simulink model "elevatorMod"  (R2020a)
settings: Solver=VariableStepAuto  StartTime=0.0  StopTime=inf  RelTol=1e-3
PreLoadFcn:
  | slplc.api.loadDataTypes;
undefined symbols (not defined in the file): BOOL, DINT, INT, slplc
libraries: simulink x1
(part 4 of 39)

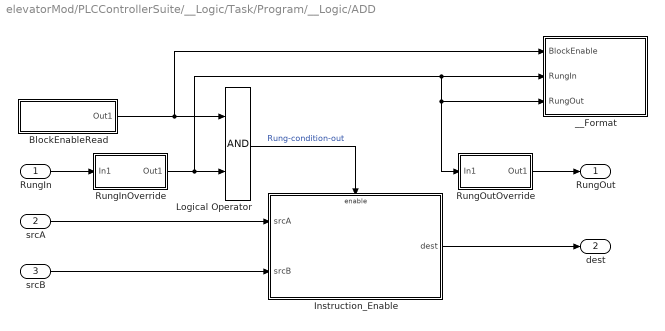
== system elevatorMod/PLCControllerSuite/__Logic/Task/Program/__Logic/ADD ==
  RungIn : Inport  OutDataTypeStr=BOOL  PortDimensions=1
  srcA : Inport  Port=2  PortDimensions=1
  srcB : Inport  Port=3  PortDimensions=1
  BlockEnableRead : Subsystem  DisableCoverage=on  TreatAsAtomicUnit=on  mask{PLCLabelTag=_Block_Enable, PLCBlockType=BlockEnableRead}
      mask prompts: PLCLabelTag "Label Tag:"
      mask init:
      | block = gcb;
      | maskObj = Simulink.Mask.get(block);
      | maskObj.Display = sprintf('disp(''%s'');', PLCLabelTag);
      mask Help: web([docroot '/plccoder/ref/blockenableread' '.html']);
      mask DialogControl PLCBlockTitle Prompt: Block Enable Read
      mask Display: disp('_Block_Enable');
  Instruction_Enable : Subsystem  TreatAsAtomicUnit=on
  Logical Operator : Logic  OutDataTypeStr=BOOL
  RungInOverride : Subsystem  DisableCoverage=on  TreatAsAtomicUnit=on
  RungOutOverride : Subsystem  DisableCoverage=on  TreatAsAtomicUnit=on
  __Format : MATLAB Function  Tag=PLC_Format_FC  Priority=20  DisableCoverage=on  InitFcn=slplc.utils.setBlockAppearance('reset');  StopFcn=slplc.utils.setBlockAppearance('reset');  TreatAsAtomicUnit=on
  RungOut : Outport  OutDataTypeStr=BOOL  PortDimensions=1  VectorParamsAs1DForOutWhenUnconnected=off
  dest : Outport  Port=2  PortDimensions=1  VectorParamsAs1DForOutWhenUnconnected=off
  wires:
  RungOutOverride/1(Out1) -> RungOut/1
  BlockEnableRead/1(Out1) -> __Format/1(BlockEnable), Logical Operator/1
  RungIn/1 -> RungInOverride/1(In1)
  RungInOverride/1(Out1) -> RungOutOverride/1(In1), __Format/3(RungOut), __Format/2(RungIn), Logical Operator/2
  srcA/1 -> Instruction_Enable/1(srcA)
  srcB/1 -> Instruction_Enable/2(srcB)
  Instruction_Enable/1(dest) -> dest/1
  Logical Operator/1 -> Instruction_Enable/Enable  "Rung-condition-out"

== system elevatorMod/PLCControllerSuite/__Logic/Task/Program/__Logic/Add Rungs ==

== system elevatorMod/PLCControllerSuite/__Logic/Task/Program/__Logic/Add Single Rung ==

== system elevatorMod/PLCControllerSuite/__Logic/Task/Program/__Logic/EQU ==
  RungIn : Inport  OutDataTypeStr=BOOL  PortDimensions=1
  srcA : Inport  Port=2  PortDimensions=1
  srcB : Inport  Port=3  PortDimensions=1
  BlockEnableRead : Subsystem  DisableCoverage=on  TreatAsAtomicUnit=on  mask{PLCLabelTag=_Block_Enable, PLCBlockType=BlockEnableRead}
      mask prompts: PLCLabelTag "Label Tag:"
      mask init:
      | block = gcb;
      | maskObj = Simulink.Mask.get(block);
      | maskObj.Display = sprintf('disp(''%s'');', PLCLabelTag);
      mask Help: web([docroot '/plccoder/ref/blockenableread' '.html']);
      mask DialogControl PLCBlockTitle Prompt: Block Enable Read
      mask Display: disp('_Block_Enable');
  Instruction_Enable : Subsystem  TreatAsAtomicUnit=on
  RungInOverride : Subsystem  DisableCoverage=on  TreatAsAtomicUnit=on
  __Format : MATLAB Function  Tag=PLC_Format_FC  Priority=20  DisableCoverage=on  InitFcn=slplc.utils.setBlockAppearance('reset');  StopFcn=slplc.utils.setBlockAppearance('reset');  TreatAsAtomicUnit=on
  RungOut : Outport  OutDataTypeStr=BOOL  PortDimensions=1  VectorParamsAs1DForOutWhenUnconnected=off
  wires:
  srcA/1 -> Instruction_Enable/2(srcA)
  Instruction_Enable/1(Rung-condition-out) -> RungOut/1, __Format/3(RungOut)
  srcB/1 -> Instruction_Enable/3(srcB)
  RungIn/1 -> RungInOverride/1(In1)
  RungInOverride/1(Out1) -> __Format/2(RungIn), Instruction_Enable/1(Rung-condition-in)
  BlockEnableRead/1(Out1) -> Instruction_Enable/Enable, __Format/1(BlockEnable)  "Rung-condition-out"

== system elevatorMod/PLCControllerSuite/__Logic/Task/Program/__Logic/EQU1 ==
  RungIn : Inport  OutDataTypeStr=BOOL  PortDimensions=1
  srcA : Inport  Port=2  PortDimensions=1
  srcB : Inport  Port=3  PortDimensions=1
  BlockEnableRead : Subsystem  DisableCoverage=on  TreatAsAtomicUnit=on  mask{PLCLabelTag=_Block_Enable, PLCBlockType=BlockEnableRead}
      mask prompts: PLCLabelTag "Label Tag:"
      mask init:
      | block = gcb;
      | maskObj = Simulink.Mask.get(block);
      | maskObj.Display = sprintf('disp(''%s'');', PLCLabelTag);
      mask Help: web([docroot '/plccoder/ref/blockenableread' '.html']);
      mask DialogControl PLCBlockTitle Prompt: Block Enable Read
      mask Display: disp('_Block_Enable');
  Instruction_Enable : Subsystem  TreatAsAtomicUnit=on
  RungInOverride : Subsystem  DisableCoverage=on  TreatAsAtomicUnit=on
  __Format : MATLAB Function  Tag=PLC_Format_FC  Priority=20  DisableCoverage=on  InitFcn=slplc.utils.setBlockAppearance('reset');  StopFcn=slplc.utils.setBlockAppearance('reset');  TreatAsAtomicUnit=on
  RungOut : Outport  OutDataTypeStr=BOOL  PortDimensions=1  VectorParamsAs1DForOutWhenUnconnected=off
  wires:
  BlockEnableRead/1(Out1) -> __Format/1(BlockEnable), Instruction_Enable/Enable  "Rung-condition-out"
  RungInOverride/1(Out1) -> Instruction_Enable/1(Rung-condition-in), __Format/2(RungIn)
  RungIn/1 -> RungInOverride/1(In1)
  srcB/1 -> Instruction_Enable/3(srcB)
  Instruction_Enable/1(Rung-condition-out) -> __Format/3(RungOut), RungOut/1
  srcA/1 -> Instruction_Enable/2(srcA)

== system elevatorMod/PLCControllerSuite/__Logic/Task/Program/__Logic/EQU2 ==
  RungIn : Inport  OutDataTypeStr=BOOL  PortDimensions=1
  srcA : Inport  Port=2  PortDimensions=1
  srcB : Inport  Port=3  PortDimensions=1
  BlockEnableRead : Subsystem  DisableCoverage=on  TreatAsAtomicUnit=on  mask{PLCLabelTag=_Block_Enable, PLCBlockType=BlockEnableRead}
      mask prompts: PLCLabelTag "Label Tag:"
      mask init:
      | block = gcb;
      | maskObj = Simulink.Mask.get(block);
      | maskObj.Display = sprintf('disp(''%s'');', PLCLabelTag);
      mask Help: web([docroot '/plccoder/ref/blockenableread' '.html']);
      mask DialogControl PLCBlockTitle Prompt: Block Enable Read
      mask Display: disp('_Block_Enable');
  Instruction_Enable : Subsystem  TreatAsAtomicUnit=on
  RungInOverride : Subsystem  DisableCoverage=on  TreatAsAtomicUnit=on
  __Format : MATLAB Function  Tag=PLC_Format_FC  Priority=20  DisableCoverage=on  InitFcn=slplc.utils.setBlockAppearance('reset');  StopFcn=slplc.utils.setBlockAppearance('reset');  TreatAsAtomicUnit=on
  RungOut : Outport  OutDataTypeStr=BOOL  PortDimensions=1  VectorParamsAs1DForOutWhenUnconnected=off
  wires:
  srcA/1 -> Instruction_Enable/2(srcA)
  Instruction_Enable/1(Rung-condition-out) -> RungOut/1, __Format/3(RungOut)
  srcB/1 -> Instruction_Enable/3(srcB)
  RungIn/1 -> RungInOverride/1(In1)
  RungInOverride/1(Out1) -> __Format/2(RungIn), Instruction_Enable/1(Rung-condition-in)
  BlockEnableRead/1(Out1) -> Instruction_Enable/Enable, __Format/1(BlockEnable)  "Rung-condition-out"

== system elevatorMod/PLCControllerSuite/__Logic/Task/Program/__Logic/EQU3 ==
  RungIn : Inport  OutDataTypeStr=BOOL  PortDimensions=1
  srcA : Inport  Port=2  PortDimensions=1
  srcB : Inport  Port=3  PortDimensions=1
  BlockEnableRead : Subsystem  DisableCoverage=on  TreatAsAtomicUnit=on  mask{PLCLabelTag=_Block_Enable, PLCBlockType=BlockEnableRead}
      mask prompts: PLCLabelTag "Label Tag:"
      mask init:
      | block = gcb;
      | maskObj = Simulink.Mask.get(block);
      | maskObj.Display = sprintf('disp(''%s'');', PLCLabelTag);
      mask Help: web([docroot '/plccoder/ref/blockenableread' '.html']);
      mask DialogControl PLCBlockTitle Prompt: Block Enable Read
      mask Display: disp('_Block_Enable');
  Instruction_Enable : Subsystem  TreatAsAtomicUnit=on
  RungInOverride : Subsystem  DisableCoverage=on  TreatAsAtomicUnit=on
  __Format : MATLAB Function  Tag=PLC_Format_FC  Priority=20  DisableCoverage=on  InitFcn=slplc.utils.setBlockAppearance('reset');  StopFcn=slplc.utils.setBlockAppearance('reset');  TreatAsAtomicUnit=on
  RungOut : Outport  OutDataTypeStr=BOOL  PortDimensions=1  VectorParamsAs1DForOutWhenUnconnected=off
  wires:
  srcA/1 -> Instruction_Enable/2(srcA)
  Instruction_Enable/1(Rung-condition-out) -> RungOut/1, __Format/3(RungOut)
  srcB/1 -> Instruction_Enable/3(srcB)
  RungIn/1 -> RungInOverride/1(In1)
  RungInOverride/1(Out1) -> __Format/2(RungIn), Instruction_Enable/1(Rung-condition-in)
  BlockEnableRead/1(Out1) -> Instruction_Enable/Enable, __Format/1(BlockEnable)  "Rung-condition-out"

== system elevatorMod/PLCControllerSuite/__Logic/Task/Program/__Logic/GRT ==
  RungIn : Inport  OutDataTypeStr=BOOL  PortDimensions=1
  srcA : Inport  Port=2  PortDimensions=1
  srcB : Inport  Port=3  PortDimensions=1
  BlockEnableRead : Subsystem  DisableCoverage=on  TreatAsAtomicUnit=on  mask{PLCLabelTag=_Block_Enable, PLCBlockType=BlockEnableRead}
      mask prompts: PLCLabelTag "Label Tag:"
      mask init:
      | block = gcb;
      | maskObj = Simulink.Mask.get(block);
      | maskObj.Display = sprintf('disp(''%s'');', PLCLabelTag);
      mask Help: web([docroot '/plccoder/ref/blockenableread' '.html']);
      mask DialogControl PLCBlockTitle Prompt: Block Enable Read
      mask Display: disp('_Block_Enable');
  Instruction_Enable : Subsystem  TreatAsAtomicUnit=on
  RungInOverride : Subsystem  DisableCoverage=on  TreatAsAtomicUnit=on
  __Format : MATLAB Function  Tag=PLC_Format_FC  Priority=20  DisableCoverage=on  InitFcn=slplc.utils.setBlockAppearance('reset');  StopFcn=slplc.utils.setBlockAppearance('reset');  TreatAsAtomicUnit=on
  RungOut : Outport  OutDataTypeStr=BOOL  PortDimensions=1  VectorParamsAs1DForOutWhenUnconnected=off
  wires:
  RungIn/1 -> RungInOverride/1(In1)
  srcB/1 -> Instruction_Enable/3(srcB)
  Instruction_Enable/1(Rung-condition-out) -> RungOut/1, __Format/3(RungOut)
  BlockEnableRead/1(Out1) -> Instruction_Enable/Enable, __Format/1(BlockEnable)
  RungInOverride/1(Out1) -> Instruction_Enable/1(Rung-condition-in), __Format/2(RungIn)
  srcA/1 -> Instruction_Enable/2(srcA)

== system elevatorMod/PLCControllerSuite/__Logic/Task/Program/__Logic/Junction ==
  RungIn1 : Inport
  RungIn2 : Inport  Port=2
  BlockEnableRead : Subsystem  DisableCoverage=on  TreatAsAtomicUnit=on  mask{PLCLabelTag=_Block_Enable, PLCBlockType=BlockEnableRead}
      mask prompts: PLCLabelTag "Label Tag:"
      mask init:
      | block = gcb;
      | maskObj = Simulink.Mask.get(block);
      | maskObj.Display = sprintf('disp(''%s'');', PLCLabelTag);
      mask Help: web([docroot '/plccoder/ref/blockenableread' '.html']);
      mask DialogControl PLCBlockTitle Prompt: Block Enable Read
      mask Display: disp('_Block_Enable');
  __Enable : Subsystem  TreatAsAtomicUnit=on
  __Format : MATLAB Function  Tag=PLC_Format_Joint  Priority=20  DisableCoverage=on  InitFcn=slplc.utils.setBlockAppearance('reset', '', {'black', 'black'});  StopFcn=slplc.utils.setBlockAppearance('reset', '', {'black', 'black'});  TreatAsAtomicUnit=on
  RungOut : Outport  VectorParamsAs1DForOutWhenUnconnected=off
  wires:
  __Enable/1(RungOut) -> RungOut/1, __Format/2(RungOut)
  RungIn2/1 -> __Enable/2(RungIn2)
  RungIn1/1 -> __Enable/1(RungIn1)
  BlockEnableRead/1(Out1) -> __Enable/Enable, __Format/1(BlockEnable)

== system elevatorMod/PLCControllerSuite/__Logic/Task/Program/__Logic/Junction1 ==
  RungIn1 : Inport
  RungIn2 : Inport  Port=2
  BlockEnableRead : Subsystem  DisableCoverage=on  TreatAsAtomicUnit=on  mask{PLCLabelTag=_Block_Enable, PLCBlockType=BlockEnableRead}
      mask prompts: PLCLabelTag "Label Tag:"
      mask init:
      | block = gcb;
      | maskObj = Simulink.Mask.get(block);
      | maskObj.Display = sprintf('disp(''%s'');', PLCLabelTag);
      mask Help: web([docroot '/plccoder/ref/blockenableread' '.html']);
      mask DialogControl PLCBlockTitle Prompt: Block Enable Read
      mask Display: disp('_Block_Enable');
  __Enable : Subsystem  TreatAsAtomicUnit=on
  __Format : MATLAB Function  Tag=PLC_Format_Joint  Priority=20  DisableCoverage=on  InitFcn=slplc.utils.setBlockAppearance('reset', '', {'black', 'black'});  StopFcn=slplc.utils.setBlockAppearance('reset', '', {'black', 'black'});  TreatAsAtomicUnit=on
  RungOut : Outport  VectorParamsAs1DForOutWhenUnconnected=off
  wires:
  BlockEnableRead/1(Out1) -> __Format/1(BlockEnable), __Enable/Enable
  RungIn1/1 -> __Enable/1(RungIn1)
  RungIn2/1 -> __Enable/2(RungIn2)
  __Enable/1(RungOut) -> __Format/2(RungOut), RungOut/1

== system elevatorMod/PLCControllerSuite/__Logic/Task/Program/__Logic/Junction10 ==
  RungIn1 : Inport
  RungIn2 : Inport  Port=2
  BlockEnableRead : Subsystem  DisableCoverage=on  TreatAsAtomicUnit=on  mask{PLCLabelTag=_Block_Enable, PLCBlockType=BlockEnableRead}
      mask prompts: PLCLabelTag "Label Tag:"
      mask init:
      | block = gcb;
      | maskObj = Simulink.Mask.get(block);
      | maskObj.Display = sprintf('disp(''%s'');', PLCLabelTag);
      mask Help: web([docroot '/plccoder/ref/blockenableread' '.html']);
      mask DialogControl PLCBlockTitle Prompt: Block Enable Read
      mask Display: disp('_Block_Enable');
  __Enable : Subsystem  TreatAsAtomicUnit=on
  __Format : MATLAB Function  Tag=PLC_Format_Joint  Priority=20  DisableCoverage=on  InitFcn=slplc.utils.setBlockAppearance('reset', '', {'black', 'black'});  StopFcn=slplc.utils.setBlockAppearance('reset', '', {'black', 'black'});  TreatAsAtomicUnit=on
  RungOut : Outport  VectorParamsAs1DForOutWhenUnconnected=off
  wires:
  __Enable/1(RungOut) -> RungOut/1, __Format/2(RungOut)
  RungIn2/1 -> __Enable/2(RungIn2)
  RungIn1/1 -> __Enable/1(RungIn1)
  BlockEnableRead/1(Out1) -> __Enable/Enable, __Format/1(BlockEnable)

== system elevatorMod/PLCControllerSuite/__Logic/Task/Program/__Logic/Junction11 ==
  RungIn1 : Inport
  RungIn2 : Inport  Port=2
  BlockEnableRead : Subsystem  DisableCoverage=on  TreatAsAtomicUnit=on  mask{PLCLabelTag=_Block_Enable, PLCBlockType=BlockEnableRead}
      mask prompts: PLCLabelTag "Label Tag:"
      mask init:
      | block = gcb;
      | maskObj = Simulink.Mask.get(block);
      | maskObj.Display = sprintf('disp(''%s'');', PLCLabelTag);
      mask Help: web([docroot '/plccoder/ref/blockenableread' '.html']);
      mask DialogControl PLCBlockTitle Prompt: Block Enable Read
      mask Display: disp('_Block_Enable');
  __Enable : Subsystem  TreatAsAtomicUnit=on
  __Format : MATLAB Function  Tag=PLC_Format_Joint  Priority=20  DisableCoverage=on  InitFcn=slplc.utils.setBlockAppearance('reset', '', {'black', 'black'});  StopFcn=slplc.utils.setBlockAppearance('reset', '', {'black', 'black'});  TreatAsAtomicUnit=on
  RungOut : Outport  VectorParamsAs1DForOutWhenUnconnected=off
  wires:
  __Enable/1(RungOut) -> RungOut/1, __Format/2(RungOut)
  RungIn2/1 -> __Enable/2(RungIn2)
  RungIn1/1 -> __Enable/1(RungIn1)
  BlockEnableRead/1(Out1) -> __Enable/Enable, __Format/1(BlockEnable)

== system elevatorMod/PLCControllerSuite/__Logic/Task/Program/__Logic/Junction12 ==
  RungIn1 : Inport
  RungIn2 : Inport  Port=2
  BlockEnableRead : Subsystem  DisableCoverage=on  TreatAsAtomicUnit=on  mask{PLCLabelTag=_Block_Enable, PLCBlockType=BlockEnableRead}
      mask prompts: PLCLabelTag "Label Tag:"
      mask init:
      | block = gcb;
      | maskObj = Simulink.Mask.get(block);
      | maskObj.Display = sprintf('disp(''%s'');', PLCLabelTag);
      mask Help: web([docroot '/plccoder/ref/blockenableread' '.html']);
      mask DialogControl PLCBlockTitle Prompt: Block Enable Read
      mask Display: disp('_Block_Enable');
  __Enable : Subsystem  TreatAsAtomicUnit=on
  __Format : MATLAB Function  Tag=PLC_Format_Joint  Priority=20  DisableCoverage=on  InitFcn=slplc.utils.setBlockAppearance('reset', '', {'black', 'black'});  StopFcn=slplc.utils.setBlockAppearance('reset', '', {'black', 'black'});  TreatAsAtomicUnit=on
  RungOut : Outport  VectorParamsAs1DForOutWhenUnconnected=off
  wires:
  BlockEnableRead/1(Out1) -> __Format/1(BlockEnable), __Enable/Enable
  RungIn1/1 -> __Enable/1(RungIn1)
  RungIn2/1 -> __Enable/2(RungIn2)
  __Enable/1(RungOut) -> __Format/2(RungOut), RungOut/1

== system elevatorMod/PLCControllerSuite/__Logic/Task/Program/__Logic/Junction13 ==
  RungIn1 : Inport
  RungIn2 : Inport  Port=2
  BlockEnableRead : Subsystem  DisableCoverage=on  TreatAsAtomicUnit=on  mask{PLCLabelTag=_Block_Enable, PLCBlockType=BlockEnableRead}
      mask prompts: PLCLabelTag "Label Tag:"
      mask init:
      | block = gcb;
      | maskObj = Simulink.Mask.get(block);
      | maskObj.Display = sprintf('disp(''%s'');', PLCLabelTag);
      mask Help: web([docroot '/plccoder/ref/blockenableread' '.html']);
      mask DialogControl PLCBlockTitle Prompt: Block Enable Read
      mask Display: disp('_Block_Enable');
  __Enable : Subsystem  TreatAsAtomicUnit=on
  __Format : MATLAB Function  Tag=PLC_Format_Joint  Priority=20  DisableCoverage=on  InitFcn=slplc.utils.setBlockAppearance('reset', '', {'black', 'black'});  StopFcn=slplc.utils.setBlockAppearance('reset', '', {'black', 'black'});  TreatAsAtomicUnit=on
  RungOut : Outport  VectorParamsAs1DForOutWhenUnconnected=off
  wires:
  __Enable/1(RungOut) -> RungOut/1, __Format/2(RungOut)
  RungIn2/1 -> __Enable/2(RungIn2)
  RungIn1/1 -> __Enable/1(RungIn1)
  BlockEnableRead/1(Out1) -> __Enable/Enable, __Format/1(BlockEnable)

== system elevatorMod/PLCControllerSuite/__Logic/Task/Program/__Logic/Junction14 ==
  RungIn1 : Inport
  RungIn2 : Inport  Port=2
  BlockEnableRead : Subsystem  DisableCoverage=on  TreatAsAtomicUnit=on  mask{PLCLabelTag=_Block_Enable, PLCBlockType=BlockEnableRead}
      mask prompts: PLCLabelTag "Label Tag:"
      mask init:
      | block = gcb;
      | maskObj = Simulink.Mask.get(block);
      | maskObj.Display = sprintf('disp(''%s'');', PLCLabelTag);
      mask Help: web([docroot '/plccoder/ref/blockenableread' '.html']);
      mask DialogControl PLCBlockTitle Prompt: Block Enable Read
      mask Display: disp('_Block_Enable');
  __Enable : Subsystem  TreatAsAtomicUnit=on
  __Format : MATLAB Function  Tag=PLC_Format_Joint  Priority=20  DisableCoverage=on  InitFcn=slplc.utils.setBlockAppearance('reset', '', {'black', 'black'});  StopFcn=slplc.utils.setBlockAppearance('reset', '', {'black', 'black'});  TreatAsAtomicUnit=on
  RungOut : Outport  VectorParamsAs1DForOutWhenUnconnected=off
  wires:
  BlockEnableRead/1(Out1) -> __Format/1(BlockEnable), __Enable/Enable
  RungIn1/1 -> __Enable/1(RungIn1)
  RungIn2/1 -> __Enable/2(RungIn2)
  __Enable/1(RungOut) -> __Format/2(RungOut), RungOut/1

== system elevatorMod/PLCControllerSuite/__Logic/Task/Program/__Logic/Junction15 ==
  RungIn1 : Inport
  RungIn2 : Inport  Port=2
  BlockEnableRead : Subsystem  DisableCoverage=on  TreatAsAtomicUnit=on  mask{PLCLabelTag=_Block_Enable, PLCBlockType=BlockEnableRead}
      mask prompts: PLCLabelTag "Label Tag:"
      mask init:
      | block = gcb;
      | maskObj = Simulink.Mask.get(block);
      | maskObj.Display = sprintf('disp(''%s'');', PLCLabelTag);
      mask Help: web([docroot '/plccoder/ref/blockenableread' '.html']);
      mask DialogControl PLCBlockTitle Prompt: Block Enable Read
      mask Display: disp('_Block_Enable');
  __Enable : Subsystem  TreatAsAtomicUnit=on
  __Format : MATLAB Function  Tag=PLC_Format_Joint  Priority=20  DisableCoverage=on  InitFcn=slplc.utils.setBlockAppearance('reset', '', {'black', 'black'});  StopFcn=slplc.utils.setBlockAppearance('reset', '', {'black', 'black'});  TreatAsAtomicUnit=on
  RungOut : Outport  VectorParamsAs1DForOutWhenUnconnected=off
  wires:
  __Enable/1(RungOut) -> RungOut/1, __Format/2(RungOut)
  RungIn2/1 -> __Enable/2(RungIn2)
  RungIn1/1 -> __Enable/1(RungIn1)
  BlockEnableRead/1(Out1) -> __Enable/Enable, __Format/1(BlockEnable)

== system elevatorMod/PLCControllerSuite/__Logic/Task/Program/__Logic/Junction16 ==
  RungIn1 : Inport
  RungIn2 : Inport  Port=2
  BlockEnableRead : Subsystem  DisableCoverage=on  TreatAsAtomicUnit=on  mask{PLCLabelTag=_Block_Enable, PLCBlockType=BlockEnableRead}
      mask prompts: PLCLabelTag "Label Tag:"
      mask init:
      | block = gcb;
      | maskObj = Simulink.Mask.get(block);
      | maskObj.Display = sprintf('disp(''%s'');', PLCLabelTag);
      mask Help: web([docroot '/plccoder/ref/blockenableread' '.html']);
      mask DialogControl PLCBlockTitle Prompt: Block Enable Read
      mask Display: disp('_Block_Enable');
  __Enable : Subsystem  TreatAsAtomicUnit=on
  __Format : MATLAB Function  Tag=PLC_Format_Joint  Priority=20  DisableCoverage=on  InitFcn=slplc.utils.setBlockAppearance('reset', '', {'black', 'black'});  StopFcn=slplc.utils.setBlockAppearance('reset', '', {'black', 'black'});  TreatAsAtomicUnit=on
  RungOut : Outport  VectorParamsAs1DForOutWhenUnconnected=off
  wires:
  BlockEnableRead/1(Out1) -> __Format/1(BlockEnable), __Enable/Enable
  RungIn1/1 -> __Enable/1(RungIn1)
  RungIn2/1 -> __Enable/2(RungIn2)
  __Enable/1(RungOut) -> __Format/2(RungOut), RungOut/1

== system elevatorMod/PLCControllerSuite/__Logic/Task/Program/__Logic/Junction17 ==
  RungIn1 : Inport
  RungIn2 : Inport  Port=2
  BlockEnableRead : Subsystem  DisableCoverage=on  TreatAsAtomicUnit=on  mask{PLCLabelTag=_Block_Enable, PLCBlockType=BlockEnableRead}
      mask prompts: PLCLabelTag "Label Tag:"
      mask init:
      | block = gcb;
      | maskObj = Simulink.Mask.get(block);
      | maskObj.Display = sprintf('disp(''%s'');', PLCLabelTag);
      mask Help: web([docroot '/plccoder/ref/blockenableread' '.html']);
      mask DialogControl PLCBlockTitle Prompt: Block Enable Read
      mask Display: disp('_Block_Enable');
  __Enable : Subsystem  TreatAsAtomicUnit=on
  __Format : MATLAB Function  Tag=PLC_Format_Joint  Priority=20  DisableCoverage=on  InitFcn=slplc.utils.setBlockAppearance('reset', '', {'black', 'black'});  StopFcn=slplc.utils.setBlockAppearance('reset', '', {'black', 'black'});  TreatAsAtomicUnit=on
  RungOut : Outport  VectorParamsAs1DForOutWhenUnconnected=off
  wires:
  __Enable/1(RungOut) -> RungOut/1, __Format/2(RungOut)
  RungIn2/1 -> __Enable/2(RungIn2)
  RungIn1/1 -> __Enable/1(RungIn1)
  BlockEnableRead/1(Out1) -> __Enable/Enable, __Format/1(BlockEnable)

== system elevatorMod/PLCControllerSuite/__Logic/Task/Program/__Logic/Junction18 ==
  RungIn1 : Inport
  RungIn2 : Inport  Port=2
  BlockEnableRead : Subsystem  DisableCoverage=on  TreatAsAtomicUnit=on  mask{PLCLabelTag=_Block_Enable, PLCBlockType=BlockEnableRead}
      mask prompts: PLCLabelTag "Label Tag:"
      mask init:
      | block = gcb;
      | maskObj = Simulink.Mask.get(block);
      | maskObj.Display = sprintf('disp(''%s'');', PLCLabelTag);
      mask Help: web([docroot '/plccoder/ref/blockenableread' '.html']);
      mask DialogControl PLCBlockTitle Prompt: Block Enable Read
      mask Display: disp('_Block_Enable');
  __Enable : Subsystem  TreatAsAtomicUnit=on
  __Format : MATLAB Function  Tag=PLC_Format_Joint  Priority=20  DisableCoverage=on  InitFcn=slplc.utils.setBlockAppearance('reset', '', {'black', 'black'});  StopFcn=slplc.utils.setBlockAppearance('reset', '', {'black', 'black'});  TreatAsAtomicUnit=on
  RungOut : Outport  VectorParamsAs1DForOutWhenUnconnected=off
  wires:
  __Enable/1(RungOut) -> RungOut/1, __Format/2(RungOut)
  RungIn2/1 -> __Enable/2(RungIn2)
  RungIn1/1 -> __Enable/1(RungIn1)
  BlockEnableRead/1(Out1) -> __Enable/Enable, __Format/1(BlockEnable)

== system elevatorMod/PLCControllerSuite/__Logic/Task/Program/__Logic/Junction19 ==
  RungIn1 : Inport
  RungIn2 : Inport  Port=2
  BlockEnableRead : Subsystem  DisableCoverage=on  TreatAsAtomicUnit=on  mask{PLCLabelTag=_Block_Enable, PLCBlockType=BlockEnableRead}
      mask prompts: PLCLabelTag "Label Tag:"
      mask init:
      | block = gcb;
      | maskObj = Simulink.Mask.get(block);
      | maskObj.Display = sprintf('disp(''%s'');', PLCLabelTag);
      mask Help: web([docroot '/plccoder/ref/blockenableread' '.html']);
      mask DialogControl PLCBlockTitle Prompt: Block Enable Read
      mask Display: disp('_Block_Enable');
  __Enable : Subsystem  TreatAsAtomicUnit=on
  __Format : MATLAB Function  Tag=PLC_Format_Joint  Priority=20  DisableCoverage=on  InitFcn=slplc.utils.setBlockAppearance('reset', '', {'black', 'black'});  StopFcn=slplc.utils.setBlockAppearance('reset', '', {'black', 'black'});  TreatAsAtomicUnit=on
  RungOut : Outport  VectorParamsAs1DForOutWhenUnconnected=off
  wires:
  __Enable/1(RungOut) -> RungOut/1, __Format/2(RungOut)
  RungIn2/1 -> __Enable/2(RungIn2)
  RungIn1/1 -> __Enable/1(RungIn1)
  BlockEnableRead/1(Out1) -> __Enable/Enable, __Format/1(BlockEnable)

== system elevatorMod/PLCControllerSuite/__Logic/Task/Program/__Logic/Junction2 ==
  RungIn1 : Inport
  RungIn2 : Inport  Port=2
  BlockEnableRead : Subsystem  DisableCoverage=on  TreatAsAtomicUnit=on  mask{PLCLabelTag=_Block_Enable, PLCBlockType=BlockEnableRead}
      mask prompts: PLCLabelTag "Label Tag:"
      mask init:
      | block = gcb;
      | maskObj = Simulink.Mask.get(block);
      | maskObj.Display = sprintf('disp(''%s'');', PLCLabelTag);
      mask Help: web([docroot '/plccoder/ref/blockenableread' '.html']);
      mask DialogControl PLCBlockTitle Prompt: Block Enable Read
      mask Display: disp('_Block_Enable');
  __Enable : Subsystem  TreatAsAtomicUnit=on
  __Format : MATLAB Function  Tag=PLC_Format_Joint  Priority=20  DisableCoverage=on  InitFcn=slplc.utils.setBlockAppearance('reset', '', {'black', 'black'});  StopFcn=slplc.utils.setBlockAppearance('reset', '', {'black', 'black'});  TreatAsAtomicUnit=on
  RungOut : Outport  VectorParamsAs1DForOutWhenUnconnected=off
  wires:
  __Enable/1(RungOut) -> RungOut/1, __Format/2(RungOut)
  RungIn2/1 -> __Enable/2(RungIn2)
  RungIn1/1 -> __Enable/1(RungIn1)
  BlockEnableRead/1(Out1) -> __Enable/Enable, __Format/1(BlockEnable)

== system elevatorMod/PLCControllerSuite/__Logic/Task/Program/__Logic/Junction20 ==
  RungIn1 : Inport
  RungIn2 : Inport  Port=2
  BlockEnableRead : Subsystem  DisableCoverage=on  TreatAsAtomicUnit=on  mask{PLCLabelTag=_Block_Enable, PLCBlockType=BlockEnableRead}
      mask prompts: PLCLabelTag "Label Tag:"
      mask init:
      | block = gcb;
      | maskObj = Simulink.Mask.get(block);
      | maskObj.Display = sprintf('disp(''%s'');', PLCLabelTag);
      mask Help: web([docroot '/plccoder/ref/blockenableread' '.html']);
      mask DialogControl PLCBlockTitle Prompt: Block Enable Read
      mask Display: disp('_Block_Enable');
  __Enable : Subsystem  TreatAsAtomicUnit=on
  __Format : MATLAB Function  Tag=PLC_Format_Joint  Priority=20  DisableCoverage=on  InitFcn=slplc.utils.setBlockAppearance('reset', '', {'black', 'black'});  StopFcn=slplc.utils.setBlockAppearance('reset', '', {'black', 'black'});  TreatAsAtomicUnit=on
  RungOut : Outport  VectorParamsAs1DForOutWhenUnconnected=off
  wires:
  __Enable/1(RungOut) -> RungOut/1, __Format/2(RungOut)
  RungIn2/1 -> __Enable/2(RungIn2)
  RungIn1/1 -> __Enable/1(RungIn1)
  BlockEnableRead/1(Out1) -> __Enable/Enable, __Format/1(BlockEnable)

== system elevatorMod/PLCControllerSuite/__Logic/Task/Program/__Logic/Junction21 ==
  RungIn1 : Inport
  RungIn2 : Inport  Port=2
  BlockEnableRead : Subsystem  DisableCoverage=on  TreatAsAtomicUnit=on  mask{PLCLabelTag=_Block_Enable, PLCBlockType=BlockEnableRead}
      mask prompts: PLCLabelTag "Label Tag:"
      mask init:
      | block = gcb;
      | maskObj = Simulink.Mask.get(block);
      | maskObj.Display = sprintf('disp(''%s'');', PLCLabelTag);
      mask Help: web([docroot '/plccoder/ref/blockenableread' '.html']);
      mask DialogControl PLCBlockTitle Prompt: Block Enable Read
      mask Display: disp('_Block_Enable');
  __Enable : Subsystem  TreatAsAtomicUnit=on
  __Format : MATLAB Function  Tag=PLC_Format_Joint  Priority=20  DisableCoverage=on  InitFcn=slplc.utils.setBlockAppearance('reset', '', {'black', 'black'});  StopFcn=slplc.utils.setBlockAppearance('reset', '', {'black', 'black'});  TreatAsAtomicUnit=on
  RungOut : Outport  VectorParamsAs1DForOutWhenUnconnected=off
  wires:
  BlockEnableRead/1(Out1) -> __Format/1(BlockEnable), __Enable/Enable
  RungIn1/1 -> __Enable/1(RungIn1)
  RungIn2/1 -> __Enable/2(RungIn2)
  __Enable/1(RungOut) -> __Format/2(RungOut), RungOut/1

== system elevatorMod/PLCControllerSuite/__Logic/Task/Program/__Logic/Junction22 ==
  RungIn1 : Inport
  RungIn2 : Inport  Port=2
  BlockEnableRead : Subsystem  DisableCoverage=on  TreatAsAtomicUnit=on  mask{PLCLabelTag=_Block_Enable, PLCBlockType=BlockEnableRead}
      mask prompts: PLCLabelTag "Label Tag:"
      mask init:
      | block = gcb;
      | maskObj = Simulink.Mask.get(block);
      | maskObj.Display = sprintf('disp(''%s'');', PLCLabelTag);
      mask Help: web([docroot '/plccoder/ref/blockenableread' '.html']);
      mask DialogControl PLCBlockTitle Prompt: Block Enable Read
      mask Display: disp('_Block_Enable');
  __Enable : Subsystem  TreatAsAtomicUnit=on
  __Format : MATLAB Function  Tag=PLC_Format_Joint  Priority=20  DisableCoverage=on  InitFcn=slplc.utils.setBlockAppearance('reset', '', {'black', 'black'});  StopFcn=slplc.utils.setBlockAppearance('reset', '', {'black', 'black'});  TreatAsAtomicUnit=on
  RungOut : Outport  VectorParamsAs1DForOutWhenUnconnected=off
  wires:
  BlockEnableRead/1(Out1) -> __Format/1(BlockEnable), __Enable/Enable
  RungIn1/1 -> __Enable/1(RungIn1)
  RungIn2/1 -> __Enable/2(RungIn2)
  __Enable/1(RungOut) -> __Format/2(RungOut), RungOut/1

== system elevatorMod/PLCControllerSuite/__Logic/Task/Program/__Logic/Junction23 ==
  RungIn1 : Inport
  RungIn2 : Inport  Port=2
  BlockEnableRead : Subsystem  DisableCoverage=on  TreatAsAtomicUnit=on  mask{PLCLabelTag=_Block_Enable, PLCBlockType=BlockEnableRead}
      mask prompts: PLCLabelTag "Label Tag:"
      mask init:
      | block = gcb;
      | maskObj = Simulink.Mask.get(block);
      | maskObj.Display = sprintf('disp(''%s'');', PLCLabelTag);
      mask Help: web([docroot '/plccoder/ref/blockenableread' '.html']);
      mask DialogControl PLCBlockTitle Prompt: Block Enable Read
      mask Display: disp('_Block_Enable');
  __Enable : Subsystem  TreatAsAtomicUnit=on
  __Format : MATLAB Function  Tag=PLC_Format_Joint  Priority=20  DisableCoverage=on  InitFcn=slplc.utils.setBlockAppearance('reset', '', {'black', 'black'});  StopFcn=slplc.utils.setBlockAppearance('reset', '', {'black', 'black'});  TreatAsAtomicUnit=on
  RungOut : Outport  VectorParamsAs1DForOutWhenUnconnected=off
  wires:
  __Enable/1(RungOut) -> RungOut/1, __Format/2(RungOut)
  RungIn2/1 -> __Enable/2(RungIn2)
  RungIn1/1 -> __Enable/1(RungIn1)
  BlockEnableRead/1(Out1) -> __Enable/Enable, __Format/1(BlockEnable)

== system elevatorMod/PLCControllerSuite/__Logic/Task/Program/__Logic/Junction24 ==
  RungIn1 : Inport
  RungIn2 : Inport  Port=2
  BlockEnableRead : Subsystem  DisableCoverage=on  TreatAsAtomicUnit=on  mask{PLCLabelTag=_Block_Enable, PLCBlockType=BlockEnableRead}
      mask prompts: PLCLabelTag "Label Tag:"
      mask init:
      | block = gcb;
      | maskObj = Simulink.Mask.get(block);
      | maskObj.Display = sprintf('disp(''%s'');', PLCLabelTag);
      mask Help: web([docroot '/plccoder/ref/blockenableread' '.html']);
      mask DialogControl PLCBlockTitle Prompt: Block Enable Read
      mask Display: disp('_Block_Enable');
  __Enable : Subsystem  TreatAsAtomicUnit=on
  __Format : MATLAB Function  Tag=PLC_Format_Joint  Priority=20  DisableCoverage=on  InitFcn=slplc.utils.setBlockAppearance('reset', '', {'black', 'black'});  StopFcn=slplc.utils.setBlockAppearance('reset', '', {'black', 'black'});  TreatAsAtomicUnit=on
  RungOut : Outport  VectorParamsAs1DForOutWhenUnconnected=off
  wires:
  __Enable/1(RungOut) -> RungOut/1, __Format/2(RungOut)
  RungIn2/1 -> __Enable/2(RungIn2)
  RungIn1/1 -> __Enable/1(RungIn1)
  BlockEnableRead/1(Out1) -> __Enable/Enable, __Format/1(BlockEnable)

== system elevatorMod/PLCControllerSuite/__Logic/Task/Program/__Logic/Junction25 ==
  RungIn1 : Inport
  RungIn2 : Inport  Port=2
  BlockEnableRead : Subsystem  DisableCoverage=on  TreatAsAtomicUnit=on  mask{PLCLabelTag=_Block_Enable, PLCBlockType=BlockEnableRead}
      mask prompts: PLCLabelTag "Label Tag:"
      mask init:
      | block = gcb;
      | maskObj = Simulink.Mask.get(block);
      | maskObj.Display = sprintf('disp(''%s'');', PLCLabelTag);
      mask Help: web([docroot '/plccoder/ref/blockenableread' '.html']);
      mask DialogControl PLCBlockTitle Prompt: Block Enable Read
      mask Display: disp('_Block_Enable');
  __Enable : Subsystem  TreatAsAtomicUnit=on
  __Format : MATLAB Function  Tag=PLC_Format_Joint  Priority=20  DisableCoverage=on  InitFcn=slplc.utils.setBlockAppearance('reset', '', {'black', 'black'});  StopFcn=slplc.utils.setBlockAppearance('reset', '', {'black', 'black'});  TreatAsAtomicUnit=on
  RungOut : Outport  VectorParamsAs1DForOutWhenUnconnected=off
  wires:
  __Enable/1(RungOut) -> RungOut/1, __Format/2(RungOut)
  RungIn2/1 -> __Enable/2(RungIn2)
  RungIn1/1 -> __Enable/1(RungIn1)
  BlockEnableRead/1(Out1) -> __Enable/Enable, __Format/1(BlockEnable)

== system elevatorMod/PLCControllerSuite/__Logic/Task/Program/__Logic/Junction26 ==
  RungIn1 : Inport
  RungIn2 : Inport  Port=2
  BlockEnableRead : Subsystem  DisableCoverage=on  TreatAsAtomicUnit=on  mask{PLCLabelTag=_Block_Enable, PLCBlockType=BlockEnableRead}
      mask prompts: PLCLabelTag "Label Tag:"
      mask init:
      | block = gcb;
      | maskObj = Simulink.Mask.get(block);
      | maskObj.Display = sprintf('disp(''%s'');', PLCLabelTag);
      mask Help: web([docroot '/plccoder/ref/blockenableread' '.html']);
      mask DialogControl PLCBlockTitle Prompt: Block Enable Read
      mask Display: disp('_Block_Enable');
  __Enable : Subsystem  TreatAsAtomicUnit=on
  __Format : MATLAB Function  Tag=PLC_Format_Joint  Priority=20  DisableCoverage=on  InitFcn=slplc.utils.setBlockAppearance('reset', '', {'black', 'black'});  StopFcn=slplc.utils.setBlockAppearance('reset', '', {'black', 'black'});  TreatAsAtomicUnit=on
  RungOut : Outport  VectorParamsAs1DForOutWhenUnconnected=off
  wires:
  BlockEnableRead/1(Out1) -> __Format/1(BlockEnable), __Enable/Enable
  RungIn1/1 -> __Enable/1(RungIn1)
  RungIn2/1 -> __Enable/2(RungIn2)
  __Enable/1(RungOut) -> __Format/2(RungOut), RungOut/1

== system elevatorMod/PLCControllerSuite/__Logic/Task/Program/__Logic/Junction27 ==
  RungIn1 : Inport
  RungIn2 : Inport  Port=2
  BlockEnableRead : Subsystem  DisableCoverage=on  TreatAsAtomicUnit=on  mask{PLCLabelTag=_Block_Enable, PLCBlockType=BlockEnableRead}
      mask prompts: PLCLabelTag "Label Tag:"
      mask init:
      | block = gcb;
      | maskObj = Simulink.Mask.get(block);
      | maskObj.Display = sprintf('disp(''%s'');', PLCLabelTag);
      mask Help: web([docroot '/plccoder/ref/blockenableread' '.html']);
      mask DialogControl PLCBlockTitle Prompt: Block Enable Read
      mask Display: disp('_Block_Enable');
  __Enable : Subsystem  TreatAsAtomicUnit=on
  __Format : MATLAB Function  Tag=PLC_Format_Joint  Priority=20  DisableCoverage=on  InitFcn=slplc.utils.setBlockAppearance('reset', '', {'black', 'black'});  StopFcn=slplc.utils.setBlockAppearance('reset', '', {'black', 'black'});  TreatAsAtomicUnit=on
  RungOut : Outport  VectorParamsAs1DForOutWhenUnconnected=off
  wires:
  BlockEnableRead/1(Out1) -> __Format/1(BlockEnable), __Enable/Enable
  RungIn1/1 -> __Enable/1(RungIn1)
  RungIn2/1 -> __Enable/2(RungIn2)
  __Enable/1(RungOut) -> __Format/2(RungOut), RungOut/1

== system elevatorMod/PLCControllerSuite/__Logic/Task/Program/__Logic/Junction28 ==
  RungIn1 : Inport
  RungIn2 : Inport  Port=2
  BlockEnableRead : Subsystem  DisableCoverage=on  TreatAsAtomicUnit=on  mask{PLCLabelTag=_Block_Enable, PLCBlockType=BlockEnableRead}
      mask prompts: PLCLabelTag "Label Tag:"
      mask init:
      | block = gcb;
      | maskObj = Simulink.Mask.get(block);
      | maskObj.Display = sprintf('disp(''%s'');', PLCLabelTag);
      mask Help: web([docroot '/plccoder/ref/blockenableread' '.html']);
      mask DialogControl PLCBlockTitle Prompt: Block Enable Read
      mask Display: disp('_Block_Enable');
  __Enable : Subsystem  TreatAsAtomicUnit=on
  __Format : MATLAB Function  Tag=PLC_Format_Joint  Priority=20  DisableCoverage=on  InitFcn=slplc.utils.setBlockAppearance('reset', '', {'black', 'black'});  StopFcn=slplc.utils.setBlockAppearance('reset', '', {'black', 'black'});  TreatAsAtomicUnit=on
  RungOut : Outport  VectorParamsAs1DForOutWhenUnconnected=off
  wires:
  __Enable/1(RungOut) -> RungOut/1, __Format/2(RungOut)
  RungIn2/1 -> __Enable/2(RungIn2)
  RungIn1/1 -> __Enable/1(RungIn1)
  BlockEnableRead/1(Out1) -> __Enable/Enable, __Format/1(BlockEnable)

== system elevatorMod/PLCControllerSuite/__Logic/Task/Program/__Logic/Junction29 ==
  RungIn1 : Inport
  RungIn2 : Inport  Port=2
  BlockEnableRead : Subsystem  DisableCoverage=on  TreatAsAtomicUnit=on  mask{PLCLabelTag=_Block_Enable, PLCBlockType=BlockEnableRead}
      mask prompts: PLCLabelTag "Label Tag:"
      mask init:
      | block = gcb;
      | maskObj = Simulink.Mask.get(block);
      | maskObj.Display = sprintf('disp(''%s'');', PLCLabelTag);
      mask Help: web([docroot '/plccoder/ref/blockenableread' '.html']);
      mask DialogControl PLCBlockTitle Prompt: Block Enable Read
      mask Display: disp('_Block_Enable');
  __Enable : Subsystem  TreatAsAtomicUnit=on
  __Format : MATLAB Function  Tag=PLC_Format_Joint  Priority=20  DisableCoverage=on  InitFcn=slplc.utils.setBlockAppearance('reset', '', {'black', 'black'});  StopFcn=slplc.utils.setBlockAppearance('reset', '', {'black', 'black'});  TreatAsAtomicUnit=on
  RungOut : Outport  VectorParamsAs1DForOutWhenUnconnected=off
  wires:
  BlockEnableRead/1(Out1) -> __Format/1(BlockEnable), __Enable/Enable
  RungIn1/1 -> __Enable/1(RungIn1)
  RungIn2/1 -> __Enable/2(RungIn2)
  __Enable/1(RungOut) -> __Format/2(RungOut), RungOut/1

== system elevatorMod/PLCControllerSuite/__Logic/Task/Program/__Logic/Junction3 ==
  RungIn1 : Inport
  RungIn2 : Inport  Port=2
  BlockEnableRead : Subsystem  DisableCoverage=on  TreatAsAtomicUnit=on  mask{PLCLabelTag=_Block_Enable, PLCBlockType=BlockEnableRead}
      mask prompts: PLCLabelTag "Label Tag:"
      mask init:
      | block = gcb;
      | maskObj = Simulink.Mask.get(block);
      | maskObj.Display = sprintf('disp(''%s'');', PLCLabelTag);
      mask Help: web([docroot '/plccoder/ref/blockenableread' '.html']);
      mask DialogControl PLCBlockTitle Prompt: Block Enable Read
      mask Display: disp('_Block_Enable');
  __Enable : Subsystem  TreatAsAtomicUnit=on
  __Format : MATLAB Function  Tag=PLC_Format_Joint  Priority=20  DisableCoverage=on  InitFcn=slplc.utils.setBlockAppearance('reset', '', {'black', 'black'});  StopFcn=slplc.utils.setBlockAppearance('reset', '', {'black', 'black'});  TreatAsAtomicUnit=on
  RungOut : Outport  VectorParamsAs1DForOutWhenUnconnected=off
  wires:
  BlockEnableRead/1(Out1) -> __Format/1(BlockEnable), __Enable/Enable
  RungIn1/1 -> __Enable/1(RungIn1)
  RungIn2/1 -> __Enable/2(RungIn2)
  __Enable/1(RungOut) -> __Format/2(RungOut), RungOut/1

== system elevatorMod/PLCControllerSuite/__Logic/Task/Program/__Logic/Junction30 ==
  RungIn1 : Inport
  RungIn2 : Inport  Port=2
  BlockEnableRead : Subsystem  DisableCoverage=on  TreatAsAtomicUnit=on  mask{PLCLabelTag=_Block_Enable, PLCBlockType=BlockEnableRead}
      mask prompts: PLCLabelTag "Label Tag:"
      mask init:
      | block = gcb;
      | maskObj = Simulink.Mask.get(block);
      | maskObj.Display = sprintf('disp(''%s'');', PLCLabelTag);
      mask Help: web([docroot '/plccoder/ref/blockenableread' '.html']);
      mask DialogControl PLCBlockTitle Prompt: Block Enable Read
      mask Display: disp('_Block_Enable');
  __Enable : Subsystem  TreatAsAtomicUnit=on
  __Format : MATLAB Function  Tag=PLC_Format_Joint  Priority=20  DisableCoverage=on  InitFcn=slplc.utils.setBlockAppearance('reset', '', {'black', 'black'});  StopFcn=slplc.utils.setBlockAppearance('reset', '', {'black', 'black'});  TreatAsAtomicUnit=on
  RungOut : Outport  VectorParamsAs1DForOutWhenUnconnected=off
  wires:
  __Enable/1(RungOut) -> RungOut/1, __Format/2(RungOut)
  RungIn2/1 -> __Enable/2(RungIn2)
  RungIn1/1 -> __Enable/1(RungIn1)
  BlockEnableRead/1(Out1) -> __Enable/Enable, __Format/1(BlockEnable)

== system elevatorMod/PLCControllerSuite/__Logic/Task/Program/__Logic/Junction31 ==
  RungIn1 : Inport
  RungIn2 : Inport  Port=2
  BlockEnableRead : Subsystem  DisableCoverage=on  TreatAsAtomicUnit=on  mask{PLCLabelTag=_Block_Enable, PLCBlockType=BlockEnableRead}
      mask prompts: PLCLabelTag "Label Tag:"
      mask init:
      | block = gcb;
      | maskObj = Simulink.Mask.get(block);
      | maskObj.Display = sprintf('disp(''%s'');', PLCLabelTag);
      mask Help: web([docroot '/plccoder/ref/blockenableread' '.html']);
      mask DialogControl PLCBlockTitle Prompt: Block Enable Read
      mask Display: disp('_Block_Enable');
  __Enable : Subsystem  TreatAsAtomicUnit=on
  __Format : MATLAB Function  Tag=PLC_Format_Joint  Priority=20  DisableCoverage=on  InitFcn=slplc.utils.setBlockAppearance('reset', '', {'black', 'black'});  StopFcn=slplc.utils.setBlockAppearance('reset', '', {'black', 'black'});  TreatAsAtomicUnit=on
  RungOut : Outport  VectorParamsAs1DForOutWhenUnconnected=off
  wires:
  __Enable/1(RungOut) -> RungOut/1, __Format/2(RungOut)
  RungIn2/1 -> __Enable/2(RungIn2)
  RungIn1/1 -> __Enable/1(RungIn1)
  BlockEnableRead/1(Out1) -> __Enable/Enable, __Format/1(BlockEnable)

== system elevatorMod/PLCControllerSuite/__Logic/Task/Program/__Logic/Junction32 ==
  RungIn1 : Inport
  RungIn2 : Inport  Port=2
  BlockEnableRead : Subsystem  DisableCoverage=on  TreatAsAtomicUnit=on  mask{PLCLabelTag=_Block_Enable, PLCBlockType=BlockEnableRead}
      mask prompts: PLCLabelTag "Label Tag:"
      mask init:
      | block = gcb;
      | maskObj = Simulink.Mask.get(block);
      | maskObj.Display = sprintf('disp(''%s'');', PLCLabelTag);
      mask Help: web([docroot '/plccoder/ref/blockenableread' '.html']);
      mask DialogControl PLCBlockTitle Prompt: Block Enable Read
      mask Display: disp('_Block_Enable');
  __Enable : Subsystem  TreatAsAtomicUnit=on
  __Format : MATLAB Function  Tag=PLC_Format_Joint  Priority=20  DisableCoverage=on  InitFcn=slplc.utils.setBlockAppearance('reset', '', {'black', 'black'});  StopFcn=slplc.utils.setBlockAppearance('reset', '', {'black', 'black'});  TreatAsAtomicUnit=on
  RungOut : Outport  VectorParamsAs1DForOutWhenUnconnected=off
  wires:
  BlockEnableRead/1(Out1) -> __Format/1(BlockEnable), __Enable/Enable
  RungIn1/1 -> __Enable/1(RungIn1)
  RungIn2/1 -> __Enable/2(RungIn2)
  __Enable/1(RungOut) -> __Format/2(RungOut), RungOut/1

== system elevatorMod/PLCControllerSuite/__Logic/Task/Program/__Logic/Junction33 ==
  RungIn1 : Inport
  RungIn2 : Inport  Port=2
  BlockEnableRead : Subsystem  DisableCoverage=on  TreatAsAtomicUnit=on  mask{PLCLabelTag=_Block_Enable, PLCBlockType=BlockEnableRead}
      mask prompts: PLCLabelTag "Label Tag:"
      mask init:
      | block = gcb;
      | maskObj = Simulink.Mask.get(block);
      | maskObj.Display = sprintf('disp(''%s'');', PLCLabelTag);
      mask Help: web([docroot '/plccoder/ref/blockenableread' '.html']);
      mask DialogControl PLCBlockTitle Prompt: Block Enable Read
      mask Display: disp('_Block_Enable');
  __Enable : Subsystem  TreatAsAtomicUnit=on
  __Format : MATLAB Function  Tag=PLC_Format_Joint  Priority=20  DisableCoverage=on  InitFcn=slplc.utils.setBlockAppearance('reset', '', {'black', 'black'});  StopFcn=slplc.utils.setBlockAppearance('reset', '', {'black', 'black'});  TreatAsAtomicUnit=on
  RungOut : Outport  VectorParamsAs1DForOutWhenUnconnected=off
  wires:
  __Enable/1(RungOut) -> RungOut/1, __Format/2(RungOut)
  RungIn2/1 -> __Enable/2(RungIn2)
  RungIn1/1 -> __Enable/1(RungIn1)
  BlockEnableRead/1(Out1) -> __Enable/Enable, __Format/1(BlockEnable)

== system elevatorMod/PLCControllerSuite/__Logic/Task/Program/__Logic/Junction34 ==
  RungIn1 : Inport
  RungIn2 : Inport  Port=2
  BlockEnableRead : Subsystem  DisableCoverage=on  TreatAsAtomicUnit=on  mask{PLCLabelTag=_Block_Enable, PLCBlockType=BlockEnableRead}
      mask prompts: PLCLabelTag "Label Tag:"
      mask init:
      | block = gcb;
      | maskObj = Simulink.Mask.get(block);
      | maskObj.Display = sprintf('disp(''%s'');', PLCLabelTag);
      mask Help: web([docroot '/plccoder/ref/blockenableread' '.html']);
      mask DialogControl PLCBlockTitle Prompt: Block Enable Read
      mask Display: disp('_Block_Enable');
  __Enable : Subsystem  TreatAsAtomicUnit=on
  __Format : MATLAB Function  Tag=PLC_Format_Joint  Priority=20  DisableCoverage=on  InitFcn=slplc.utils.setBlockAppearance('reset', '', {'black', 'black'});  StopFcn=slplc.utils.setBlockAppearance('reset', '', {'black', 'black'});  TreatAsAtomicUnit=on
  RungOut : Outport  VectorParamsAs1DForOutWhenUnconnected=off
  wires:
  __Enable/1(RungOut) -> RungOut/1, __Format/2(RungOut)
  RungIn2/1 -> __Enable/2(RungIn2)
  RungIn1/1 -> __Enable/1(RungIn1)
  BlockEnableRead/1(Out1) -> __Enable/Enable, __Format/1(BlockEnable)

== system elevatorMod/PLCControllerSuite/__Logic/Task/Program/__Logic/Junction35 ==
  RungIn1 : Inport
  RungIn2 : Inport  Port=2
  BlockEnableRead : Subsystem  DisableCoverage=on  TreatAsAtomicUnit=on  mask{PLCLabelTag=_Block_Enable, PLCBlockType=BlockEnableRead}
      mask prompts: PLCLabelTag "Label Tag:"
      mask init:
      | block = gcb;
      | maskObj = Simulink.Mask.get(block);
      | maskObj.Display = sprintf('disp(''%s'');', PLCLabelTag);
      mask Help: web([docroot '/plccoder/ref/blockenableread' '.html']);
      mask DialogControl PLCBlockTitle Prompt: Block Enable Read
      mask Display: disp('_Block_Enable');
  __Enable : Subsystem  TreatAsAtomicUnit=on
  __Format : MATLAB Function  Tag=PLC_Format_Joint  Priority=20  DisableCoverage=on  InitFcn=slplc.utils.setBlockAppearance('reset', '', {'black', 'black'});  StopFcn=slplc.utils.setBlockAppearance('reset', '', {'black', 'black'});  TreatAsAtomicUnit=on
  RungOut : Outport  VectorParamsAs1DForOutWhenUnconnected=off
  wires:
  BlockEnableRead/1(Out1) -> __Format/1(BlockEnable), __Enable/Enable
  RungIn1/1 -> __Enable/1(RungIn1)
  RungIn2/1 -> __Enable/2(RungIn2)
  __Enable/1(RungOut) -> __Format/2(RungOut), RungOut/1

== system elevatorMod/PLCControllerSuite/__Logic/Task/Program/__Logic/Junction4 ==
  RungIn1 : Inport
  RungIn2 : Inport  Port=2
  BlockEnableRead : Subsystem  DisableCoverage=on  TreatAsAtomicUnit=on  mask{PLCLabelTag=_Block_Enable, PLCBlockType=BlockEnableRead}
      mask prompts: PLCLabelTag "Label Tag:"
      mask init:
      | block = gcb;
      | maskObj = Simulink.Mask.get(block);
      | maskObj.Display = sprintf('disp(''%s'');', PLCLabelTag);
      mask Help: web([docroot '/plccoder/ref/blockenableread' '.html']);
      mask DialogControl PLCBlockTitle Prompt: Block Enable Read
      mask Display: disp('_Block_Enable');
  __Enable : Subsystem  TreatAsAtomicUnit=on
  __Format : MATLAB Function  Tag=PLC_Format_Joint  Priority=20  DisableCoverage=on  InitFcn=slplc.utils.setBlockAppearance('reset', '', {'black', 'black'});  StopFcn=slplc.utils.setBlockAppearance('reset', '', {'black', 'black'});  TreatAsAtomicUnit=on
  RungOut : Outport  VectorParamsAs1DForOutWhenUnconnected=off
  wires:
  __Enable/1(RungOut) -> RungOut/1, __Format/2(RungOut)
  RungIn2/1 -> __Enable/2(RungIn2)
  RungIn1/1 -> __Enable/1(RungIn1)
  BlockEnableRead/1(Out1) -> __Enable/Enable, __Format/1(BlockEnable)

== system elevatorMod/PLCControllerSuite/__Logic/Task/Program/__Logic/Junction5 ==
  RungIn1 : Inport
  RungIn2 : Inport  Port=2
  BlockEnableRead : Subsystem  DisableCoverage=on  TreatAsAtomicUnit=on  mask{PLCLabelTag=_Block_Enable, PLCBlockType=BlockEnableRead}
      mask prompts: PLCLabelTag "Label Tag:"
      mask init:
      | block = gcb;
      | maskObj = Simulink.Mask.get(block);
      | maskObj.Display = sprintf('disp(''%s'');', PLCLabelTag);
      mask Help: web([docroot '/plccoder/ref/blockenableread' '.html']);
      mask DialogControl PLCBlockTitle Prompt: Block Enable Read
      mask Display: disp('_Block_Enable');
  __Enable : Subsystem  TreatAsAtomicUnit=on
  __Format : MATLAB Function  Tag=PLC_Format_Joint  Priority=20  DisableCoverage=on  InitFcn=slplc.utils.setBlockAppearance('reset', '', {'black', 'black'});  StopFcn=slplc.utils.setBlockAppearance('reset', '', {'black', 'black'});  TreatAsAtomicUnit=on
  RungOut : Outport  VectorParamsAs1DForOutWhenUnconnected=off
  wires:
  BlockEnableRead/1(Out1) -> __Format/1(BlockEnable), __Enable/Enable
  RungIn1/1 -> __Enable/1(RungIn1)
  RungIn2/1 -> __Enable/2(RungIn2)
  __Enable/1(RungOut) -> __Format/2(RungOut), RungOut/1

== system elevatorMod/PLCControllerSuite/__Logic/Task/Program/__Logic/Junction6 ==
  RungIn1 : Inport
  RungIn2 : Inport  Port=2
  BlockEnableRead : Subsystem  DisableCoverage=on  TreatAsAtomicUnit=on  mask{PLCLabelTag=_Block_Enable, PLCBlockType=BlockEnableRead}
      mask prompts: PLCLabelTag "Label Tag:"
      mask init:
      | block = gcb;
      | maskObj = Simulink.Mask.get(block);
      | maskObj.Display = sprintf('disp(''%s'');', PLCLabelTag);
      mask Help: web([docroot '/plccoder/ref/blockenableread' '.html']);
      mask DialogControl PLCBlockTitle Prompt: Block Enable Read
      mask Display: disp('_Block_Enable');
  __Enable : Subsystem  TreatAsAtomicUnit=on
  __Format : MATLAB Function  Tag=PLC_Format_Joint  Priority=20  DisableCoverage=on  InitFcn=slplc.utils.setBlockAppearance('reset', '', {'black', 'black'});  StopFcn=slplc.utils.setBlockAppearance('reset', '', {'black', 'black'});  TreatAsAtomicUnit=on
  RungOut : Outport  VectorParamsAs1DForOutWhenUnconnected=off
  wires:
  __Enable/1(RungOut) -> RungOut/1, __Format/2(RungOut)
  RungIn2/1 -> __Enable/2(RungIn2)
  RungIn1/1 -> __Enable/1(RungIn1)
  BlockEnableRead/1(Out1) -> __Enable/Enable, __Format/1(BlockEnable)
